simulink model "mobileSim"  (R2013b)
settings: Solver=ode4  StartTime=0.0  StopTime=0.05  FixedStep=0.05  RelTol=1e-3
values from neighbouring files (symbols this model uses):
  omegaL = sum(wL)/5    [RunSim.m]
  omegaR = sum(wR)/5    [RunSim.m]
undefined symbols (not defined in the file): fi_1, x_1, y_1
settings Model: Creator=Nezir  LastModifiedBy=Nezir

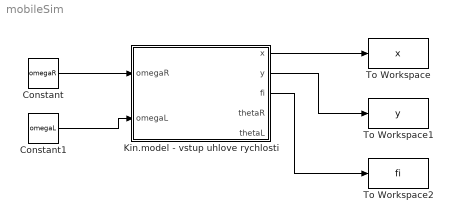
== system mobileSim ==
  Constant : Constant  Value=omegaR
  Constant1 : Constant  Value=omegaL
  Kin.model - vstup uhlove rychlosti : Subsystem  mask{L=0.068, r=0.024, x=x_1, y=y_1, fi=fi_1}
      mask prompts: L "L - rozchod kolies [m]"; r "r - polomer kolesa [m]"; x "x - pociatocna podmienka"; y "y - pociatocna podmienka"; fi "fi - pociatocna podmienka"
      mask Help: http://neuron.tuke.sk/klein/Bakalarka/kin_model_uhlove_rychlosti.pdf
      mask Display:
      | port_label('input', 1, '\it \omega_R(t)','interpreter','tex')
      | port_label('input', 2, '\it \omega_L(t)','interpreter','tex')
      | port_label('output', 1, '\it x(t)','interpreter','tex')
      | port_label('output', 2, '\it y(t)','interpreter','tex')
      | port_label('output', 3, '\it \phi(t)','interpreter','tex')
      | port_label('output', 4, '\it \theta_R(t)','interpreter','tex')
      | port_label('output', 5, '\it \theta_L(t)','interpreter','tex')
      | fprintf('Kinematický model')
  To Workspace : ToWorkspace  VariableName=x  SampleTime=-1
  To Workspace1 : ToWorkspace  VariableName=y  SampleTime=-1
  To Workspace2 : ToWorkspace  VariableName=fi  SampleTime=-1
  wires:
  Kin.model - vstup uhlove rychlosti/1(x) -> To Workspace/1
  Kin.model - vstup uhlove rychlosti/2(y) -> To Workspace1/1
  Kin.model - vstup uhlove rychlosti/3(fi) -> To Workspace2/1
  Constant/1 -> Kin.model - vstup uhlove rychlosti/1(omegaR)
  Constant1/1 -> Kin.model - vstup uhlove rychlosti/2(omegaL)

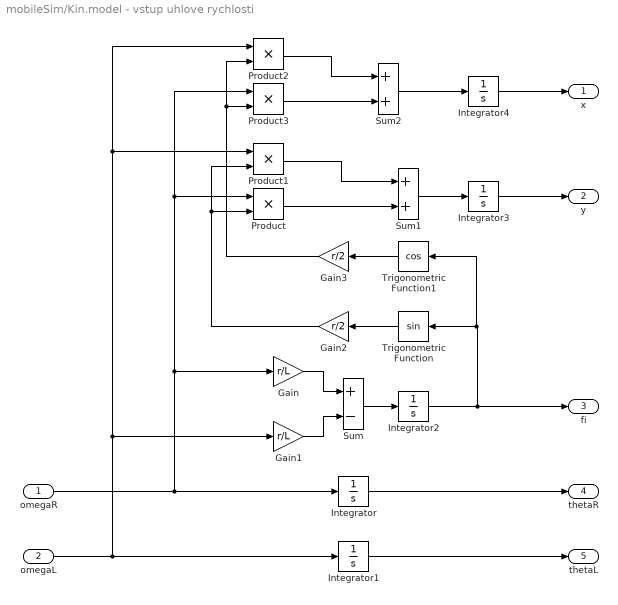
== system mobileSim/Kin.model - vstup uhlove rychlosti ==
  omegaR : Inport
  omegaL : Inport  Port=2
  Gain : Gain  Gain=r/L
  Gain1 : Gain  Gain=r/L
  Gain2 : Gain  Gain=r/2
  Gain3 : Gain  Gain=r/2
  Integrator : Integrator
  Integrator1 : Integrator
  Integrator2 : Integrator  InitialCondition=fi
  Integrator3 : Integrator  InitialCondition=y
  Integrator4 : Integrator  InitialCondition=x
  Product{,1..3} (4 alike) : Product
  Sum : Sum  Inputs=+-
  Sum1 : Sum
  Sum2 : Sum
  Trigonometric Function : Trigonometry
  Trigonometric Function1 : Trigonometry  Operator=cos
  x : Outport
  y : Outport  Port=2
  fi : Outport  Port=3
  thetaR : Outport  Port=4
  thetaL : Outport  Port=5
  wires:
  Integrator4/1 -> x/1
  Gain3/1 -> Product2/2, Product3/2
  Product3/1 -> Sum2/2
  Gain2/1 -> Product/2, Product1/2
  Product2/1 -> Sum2/1
  Product1/1 -> Sum1/1
  Product/1 -> Sum1/2
  Trigonometric Function/1 -> Gain2/1
  Sum2/1 -> Integrator4/1
  Trigonometric Function1/1 -> Gain3/1
  Integrator3/1 -> y/1
  Integrator/1 -> thetaR/1
  omegaR/1 -> Product/1, Product3/1, Gain/1, Integrator/1
  Integrator1/1 -> thetaL/1
  omegaL/1 -> Product1/1, Product2/1, Gain1/1, Integrator1/1
  Gain1/1 -> Sum/2
  Integrator2/1 -> Trigonometric Function/1, Trigonometric Function1/1, fi/1
  Sum1/1 -> Integrator3/1
  Sum/1 -> Integrator2/1
  Gain/1 -> Sum/1
